simulink model "sim_Motorl"  (Simulink 7.5)
settings: Solver=ode3  StartTime=0.0  StopTime=1  RelTol=1e-4
undefined symbols (not defined in the file or in its folder): level
libraries: powerlib x8, powerlib_extras x3
settings Model: Creator=Kun Zhang  LastModifiedBy=Kun Zhang

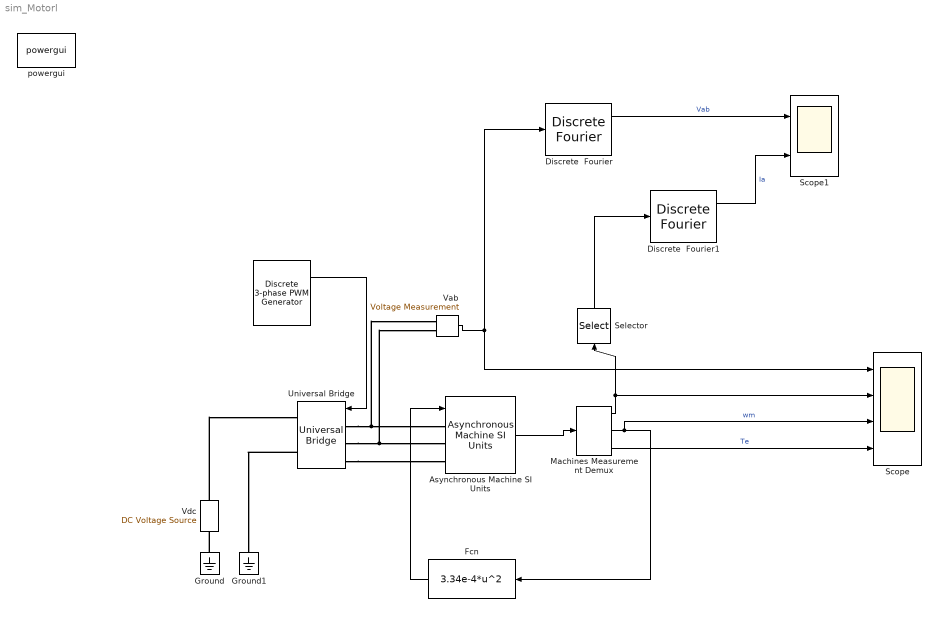
== system sim_Motorl ==
  " " : powerlib_extras/Discrete  Control Blocks/Discrete 3-phase PWM Generator  DialogController=POWERSYS.PowerSysDialog  SystemSampleTime=-1  ModulatorType=3-level  ModulatorMode=Un-synchronized  nF=18  Fc=18*60  ModulatingSignals=on  m=0.9  Freq=50  Phase=0  Ts=10e-6
  Asynchronous Machine SI Units : powerlib/Machines/Asynchronous Machine SI Units  DialogController=POWERSYS.PowerSysDialog  SystemSampleTime=-1  PresetModel=No  MechanicalLoad=Torque Tm  ShowDetailedParameters=on  RotorType=Squirrel-cage  ReferenceFrame=Rotor  NominalParameters=[ 3*746, 220, 60 ]  Stator=[ 1.115 0.005974]  Rotor=[ 1.083 0.005974]  Lm=0.2037  Mechanical=[0.02 0.005752 2]  PolePairs=2  InitialConditions=[1 0 0 0 0 0 0 0]  Units=SI  LoadFlowParameters=1492000  SimulateSaturation=off  Saturation=[14.03593122, 27.81365428, 53.79336849, 72.68890987, 97.98006896, 148.6815601, 215.7428561, 302.9841135, 428.7778367 ; 230, 322, 414, 460, 506, 552, 598, 644, 690]  TsPowergui=0  TsBlock=-1  IterativeModel=Forward Euler
  Discrete  Fourier : powerlib_extras/Discrete Measurements/Discrete  Fourier  DialogController=POWERSYS.PowerSysDialog  SystemSampleTime=-1  Freq=60  n=1  Par_Init=[0 0]  Ts=10e-6
  Discrete  Fourier1 : powerlib_extras/Discrete Measurements/Discrete  Fourier  DialogController=POWERSYS.PowerSysDialog  SystemSampleTime=-1  Freq=60  n=1  Par_Init=[0 0]  Ts=10e-6
  Fcn : Fcn  Expr=3.34e-4*u^2
  Ground : powerlib/Elements/Ground  DialogController=POWERSYS.PowerSysDialog  PhysicalDomain=powersysdomain  SubClassName=unknown  LeftPortType=p1  RightPortType=p1  LConnTagsString=a
  Ground1 : powerlib/Elements/Ground  DialogController=POWERSYS.PowerSysDialog  PhysicalDomain=powersysdomain  SubClassName=unknown  LeftPortType=p1  RightPortType=p1  LConnTagsString=a
  Machines Measurement Demux : powerlib/Machines/Machines Measurement Demux  DialogController=POWERSYS.PowerSysDialog  SystemSampleTime=-1  machType=Asynchronous  ssm1=on  ssm2=on  ssm3=on  ssm4=on  ssm5=on  ssm6=on  sm1=off  sm2=off  sm3=off  sm4=off  sm5=off  sm6=off  sm7=off  sm8=on  sm9=off  sm10=off  sm11=off  sm115=off  sm12=off  sm13=off  sm14=off  asm1=off  asm2=off  asm3=off  asm4=off  asm5=on  asm6=off  asm7=off  asm8=off  asm9=on  asm10=on  asm11=off  pmsm1=on  pmsm2=on  pmsm3=on  pmsm4=off  pmsm5=on  pmsm6=on  pmsm7=on  lastType=1
  Scope : Scope  NumInputPorts=4
      settings: TimeRange=0.05  YMin=-5~-5~-5~-5  YMax=5~5~5~5  SaveName=ASM
  Scope1 : Scope  NumInputPorts=2
      settings: TimeRange=0.05  YMin=-5~-5  YMax=5~5  SaveName=ASM1
  Selector : Selector  InputPortWidth=3  IndexOptions=Index vector (dialog)  Indices=1  OutputSizes=1
  Universal Bridge : powerlib/Power Electronics/Universal Bridge  DialogController=POWERSYS.PowerSysDialog  SystemSampleTime=-1  Arms=3  SnubberResistance=1e5  SnubberCapacitance=inf  Device=IGBT / Diodes  Ron=1e-3  Lon=0  ForwardVoltages="[  0  0  ]"  ForwardVoltage=0  GTOparameters=[ 10e-6 , 20e-6 ]  IGBTparameters=[ 1e-6 , 1e-6 ]  Measurements=None  Measurements_2=None  converterType=Rectifier
  Vab : powerlib/Measurements/Voltage Measurement  DialogController=POWERSYS.PowerSysDialog  SystemSampleTime=-1  PhasorSimulation=off  OutputType=Complex  PSBequivalent=0
  Vdc : powerlib/Electrical Sources/DC Voltage Source  DialogController=POWERSYS.PowerSysDialog  SystemSampleTime=-1  Amplitude=514  Measurements=None
  powergui : powerlib/powergui  Priority=1  SystemSampleTime=-1  SimulationMode=Discrete  SampleTime=10e-6  frequency=60  SPID=off  DisableSnubberDevices=off  DisableRonSwitches=off  DisableVfSwitches=off  SwTol=0  Interpol=off  frequencyindice=60  echomessages=off  HookPort=off  DisplayEquations=off  FunctionMessages=off  EnableUseOfTLC=off  x0status=blocks  RestoreLinks=warning  ResistiveCurrentMeasurement=off  Ylog=off  Xlog=on  ShowGrid=off  save=off  variable=ZData  structure=ASM1  ZoomFFT=off  StartTime=0  cycles=20  DisplayStyle=1  fundamental=60  FreqAxis=on  MaxFrequency=5000  frequencyindicesteady=1  display=off  methode=off
  wires:
  Fcn/1 -> Asynchronous Machine SI Units/1
  Machines Measurement Demux/2 -> Fcn/1, Scope/3  "wm"
  " "/1 -> Universal Bridge/1
  Vab/1 -> Scope/1, Discrete  Fourier/1
  Selector/1 -> Discrete  Fourier1/1
  Machines Measurement Demux/1 -> Selector/1, Scope/2
  Machines Measurement Demux/3 -> Scope/4  "Te"
  Asynchronous Machine SI Units/1 -> Machines Measurement Demux/1
  Discrete  Fourier1/1 -> Scope1/2  "Ia"
  Discrete  Fourier/1 -> Scope1/1  "Vab"
  connections:
  Ground/LConn1 -- Vdc/LConn1
  Universal Bridge/LConn1 -- Asynchronous Machine SI Units/LConn1 -- Vab/LConn1
  Universal Bridge/LConn2 -- Asynchronous Machine SI Units/LConn2 -- Vab/LConn2
  Vdc/RConn1 -- Universal Bridge/RConn1
  Universal Bridge/RConn2 -- Ground1/LConn1
  Universal Bridge/LConn3 -- Asynchronous Machine SI Units/LConn3
